simulink model "LQR_ACC_research"  (R2024a)
settings: Solver=FixedStepAuto  StartTime=0  StopTime=100  FixedStep=0.05  RelTol=1e-3
undefined symbols (not defined in the file or in its folder): acc_max, acc_min, Defined, driver_set_speed, Ego, jerk_lim, K_derr, K_vh, Lane, matlabshared, rho, simStepSize, User
libraries: roadrunnerscenario x5, dsa_UDP_Blockset x2, autolibshared x1, drivingscenarioandsensors x1
settings Model: PacingRate=10  Creator=darkh  LastModifiedBy=darkh
settings DataIOCC: ReturnWorkspaceOutputsName=sltest_internal_rrSimulationOutputVariable
settings DebuggingCC: AlgebraicLoopMsg=none
settings RTWCC: GPUComputeCapability=3.5
settings ConfigComp: CovSaveName=sltest_covdata  CovMetricSettings=dcmwe  CovEnableCumulative=off  CovSaveSingleToWorkspaceVar=on  CovSaveOutputData=off

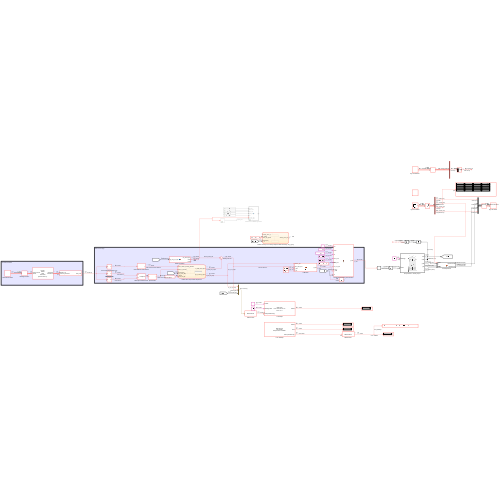
[thumbnail: Simulink's stored preview of the top-level diagram]
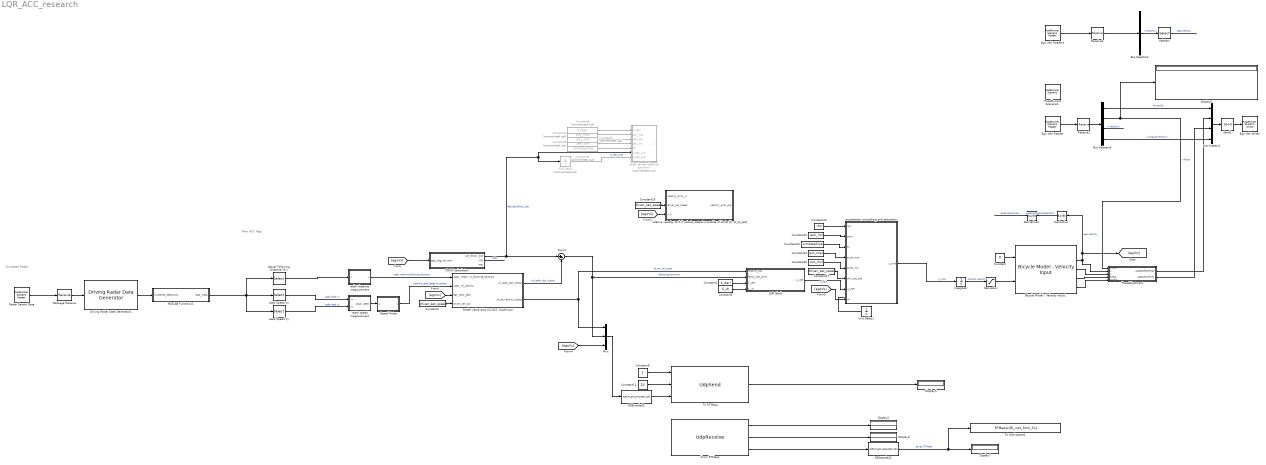
== system LQR_ACC_research ==
  note: Simulated Radar
  note: Main ACC Algo
  Actual Following Distance (dx) : Selector  InputPortWidth=6  IndexOptions=Index vector (dialog)  Indices=[1]  OutputSizes=1
  Bicycle Model - Velocity Input1 : autolibshared/Bicycle Model - Velocity Input  trackMode=Single (bicycle)  inputMode=External longitudinal velocity  frontSteerMode=on  rearSteerMode=off  windMode=off  muMode=off  extFMode=off  extMMode=off  aMode=3  NF=2  NR=2  m=2630.84  a=1.2  b=1.6  h=0.35  X_o=0  xdot_o=0  CalphaMode=off  sigmaMode=on  w=[1.4,1.4]  Cy_f=19000  Cy_r=33000  sigma_f=.1  sigma_r=.1  alpha_f_brk=[-.1 .1]  Cy_f_data=[-9e3 9e3]  alpha_r_brk=[-.1 .1]  Cy_r_data=[-9e3 9e3]  Y_o=0  ydot_o=0  Izz=2875  psi_o=0  r_o=0  Af=2  Cd=.3  Cl=.1  Cpm=.1  beta_w=[0 0.01:0.01:0.3]  Cs=[0 0.01:0.01:0.3]  Cym=[0 1e-6:0.01:0.3]  Pabs=101325  Tair=273  g=9.81  mu=1  xdot_tol=.01  Fznom=5000  Fxtire_sat=1e6  Fytire_sat=1e6  longOff=0  latOff=0  vertOff=0
      settings: LibrarySourceBlock=drivingscenarioandsensors/Bicycle Model - Velocity Input
  Bus Creator1 : BusCreator  Inputs=4  OutDataTypeStr=Bus: BusActorRuntime  NonVirtualBus=on
      settings: InheritFromInputs=off
  Bus Selector1 : BusSelector  OutputSignals=ActorRuntime.Velocity
  Bus Selector3 : BusSelector  OutputSignals=ActorID,Pose,Velocity,AngularVelocity
  Constant : Constant  Value=0
  Constant1 : Constant  Value=K_derr  SampleTime=simStepSize
  Constant10 : Constant  Value=rho
  Constant11 : Constant  Value=24
  Constant12 : Constant  Value=jerk_lim
  Constant13 : Constant  Value=simStepSize
  Constant14 : Constant  Value=acc_max
  Constant15 : Constant  Value=acc_min
  Constant16 : Constant  Value=driver_set_speed  SampleTime=simStepSize
  Constant17 : Constant  Value=driver_set_speed  SampleTime=simStepSize
  Constant2 : Constant  Value=driver_set_speed  SampleTime=simStepSize
  Constant3 : Constant  Value=K_vh  SampleTime=simStepSize
  Constant4 : Constant  Commented=on  Value=simStepSize
  Constant5 : Constant  Commented=on  Value=jerk_lim
  Constant6 : Constant  Commented=on  Value=acc_min
  Constant7 : Constant  Commented=on  Value=acc_max
  Constant8 : Constant  Commented=on  Value=K_derr
  Constant9 : Constant
  "DSDecode32 " : S-Function  FunctionName=ds867c_eth_decode32_sfcn  Parameters=byteordering,offset,auto_offset,datatype,one_datatype,sampletime  SFunctionDeploymentMode=off  EnableBusSupport=off  mask(DSDecode32){byteordering=big endian (Motorola), offset=[0], auto_offset=on, datatype=[9], one_datatype=off, sampletime=-1}
      mask prompts: byteordering "Byte ordering:"; offset "Offset (bytes):"; auto_offset "Auto offset"; one_datatype "One datatype only"
      mask help:
      | Converts a 32bit WORD input data stream into the specified datatypes on the output port.
      |
      | Datatype Codes:
      | BOOLEAN:  1   //   INT8      :  2    //   UINT8    :  3
      | INT16       :  4   //   UINT16 :  5    //   INT32     :  6
      | UINT32    :  7   //   FLOAT   :  8    //   DOUBLE:  9
      mask Help:
      | The 'DSDecode32' block allows to decode an UInt32 vector containing encoded elements of various data types to an output vector of double values. It is intended to use this block in conjunction with the 'DS4504_ETH_Receive' block which delivers this format as data output. Data received from the Ethernet via the 'DS4504_ETH_Receive' block is performed in Intel byte order ('Little Endian').
      | 
      | <br>
      | <br>
      | 
      | <h2>Parameters</h2>
      | <br>
      | <br>
      | 
      | <b>Byte ordering (only relevant for offline simulation)</b>
      | <br>
      | <blockquote>
      | The byte order of the input vector has to be specified. In case of running a real-time application the appropriate byte order (Motorola for DS1005 and Intel for DS1006) is selected automatically. Therefore the byte order setting has no influence on the online simulation.
      | </blockquote>
      | <br>
      | 
      | <b>Offset (bytes)</b>
      | <br>
      | <blockquote>
      | This is for defining a vector of offsets which specifies the position of each element within the input vector. The offsets must be entered as an array (e.g. [1 10 . 50 54] ) using the same order as for the corresponding data type vector (see (4)). This option is useful if you have gaps between adjacent elements.
      | </blockquote>
      | <br>
      | 
      | <b>Auto offset</b>
      | <br>
      | <blockquote>
      | When activating this checkbox parameter, the edit field 'Offset' is disabled and the byte offsets in the input vector are calculated automatically concerning the specified data types (no gaps presupposed). Any previous setting in the offset vector would be ignored.
      | </blockquote>
      | <br>
      | 
      | <b>Datatype</b>
      | <br>
      | <blockquote>
      | This is for defining a vector of data types which specifies the type for each element in the input vector. Supported data types are Boolean, Int8, UInt8, Int16, UInt16, Int32, UInt32, Float and Double, which are determined by using the corresponding data type codes shown in the following table:
      | <br>
      | <br>
      | <table BORDER=1 ALIGN="center">
      | <TR>
      | <TH WIDTH=20%>Data type</TH>
      | <TH WIDTH=20%>Data type code</TH>
      | <TH WIDTH=20%>Length in bytes</TH>
      | </TR>
      | <TR><TD>Boolean</TD><TD ALIGN="center">1</TD><TD ALIGN="center">1</TD></TR>
      | <TR><TD>Int8</TD><TD ALIGN="center">2</TD><TD ALIGN="center">1</TD></TR>
      | <TR><TD>Uint8</TD><TD ALIGN="center">3</TD><TD ALIGN="center">1</TD></TR>
      | <TR><TD>Int16</TD><TD ALIGN="center">4</TD><TD ALIGN="center">2</TD></TR>
      | <TR><TD>Uint16</TD><TD ALIGN="center">5</TD><TD ALIGN="center">2</TD></TR>
      | <TR><TD>Int32</TD><TD ALIGN="center">6</TD><TD ALIGN="center">4</TD></TR>
      | <TR><TD>Uint32</TD><TD ALIGN="center">7</TD><TD ALIGN="center">4</TD></TR>
      | <TR><TD>Float</TD><TD ALIGN="center">8</TD><TD ALIGN="center">4</TD></TR>
      | <TR><TD>Double</TD><TD ALIGN="center">9</TD><TD ALIGN="center">8</TD></TR>
      | </TABLE>
      | </blockquote>
      | <br>
      | 
      | <b>One datatype only</b>
      | <br>
      | <blockquote>
      | This option is useful if all elements of the input vector have the same data type. If the checkbox is activated the first element of the data type vector specifies the data type to be used. In this case it is naturally sufficient to enter only one number which applies for the complete input vector.
      | </blockquote>
      | <br>
      | 
      | <b>Sample time</b>
      | <br>
      | <blockquote>
      | The desired sample time for this block has to be entered here. Alternatively it can be  inherited from the Simulink model by using '-1'.
      | </blockquote>
      | <br>
      mask TypeOptions byteordering: big endian (Motorola) | little endian (Intel)
      mask Display: text(0.5,0.5,'DSDecode32','HorizontalAlignment','center')
  DSEncode32 : S-Function  FunctionName=ds867c_eth_encode32_sfcn  Parameters=byteordering,offset,auto_offset,datatype,one_datatype,sampletime  SFunctionDeploymentMode=off  EnableBusSupport=off  mask(DSEncode32){byteordering=big endian (Motorola), offset=[ 0 ], auto_offset=on, datatype=[9,9,9], one_datatype=off, sampletime=-1}
      mask prompts: byteordering "Byte ordering:"; offset "Offset (bytes):"; auto_offset "Auto offset"; one_datatype "One datatype only"
      mask help:
      | Converts an input signal consisting of datatypes into a 32Bit WORD data stream on the output port.
      |
      | Datatype Codes:
      | BOOLEAN:  1   //   INT8      :  2    //   UINT8    :  3
      | INT16       :  4   //   UINT16 :  5    //   INT32     :  6
      | UINT32    :  7   //   FLOAT   :  8    //   DOUBLE:  9
      mask Help:
      | The 'DSEncode32' block is responsible for converting the input vector consisting of double values to different data types (multi-byte numbers) and merging them into a data stream composed of an array of UInt32 variables. It is intended to use this block in conjunction with the 'DS4504_ETH_Send' block which delivers the data in Intel byte order to the network.
      | 
      | <br>
      | <br>
      | 
      | <h2>Parameters</h2>
      | <br>
      | <br>
      | 
      | <b>Byte ordering (only relevant for offline simulation)</b>
      | <br>
      | <blockquote>
      | It lets the user choose the byte order (Motorola or Intel) of the output vector. The way multibyte numbers (e.g. Float = 4 bytes or Int16 = 2 bytes) are stored in memory depends on the used computing system. There are two possible formats which are called "Little Endian" and "Big Endian". "Little Endian" means that the low-order byte of the number is stored at the lowest and the high-order byte at the highest memory address. "Big Endian" means the opposite.
      | This option is only relevant for offline (Simulink) simulation. In case of running a real-time application the appropriate byte order (Motorola for DS1005 and Intel for DS1006) is selected automatically. Therefore the byte order setting has no influence on the online simulation.
      | </blockquote>
      | <br>
      | 
      | <b>Offset (bytes)</b>
      | <br>
      | <blockquote>
      | This is for defining a vector of offsets which specifies the position of each input element within the output byte vector. The offsets must be entered as an array (e.g. [1 10 . 50 54] ) using the same order as for the corresponding data type vector (see (4)). This option is useful if you want to have gaps between adjacent elements (e.g. in order to avoid access to even bytes).
      | <br>
      | <br>
      | <i>Important Note:</i>
      | <br>
      | By means of the offset vector the specified data values can be located flexibly within the UInt32 word stream, presupposed that the data values do not overlap. Otherwise data loss occurs.
      | </blockquote>
      | <br>
      | 
      | <b>Auto offset</b>
      | <br>
      | <blockquote>
      | When activating this checkbox parameter, the edit field 'Offset' is disabled and the required byte offsets for the input data types will be calculated automatically without gaps (for tight packing). This option is always useful if there is no need for special offsets (no gaps between two adjacent elements). Any previous setting in the offset vector would be ignored.
      | </blockquote>
      | <br>
      | 
      | <b>Datatype</b>
      | <br>
      | <blockquote>
      | This is for defining a vector of data types which specifies the type for each input element in the output byte vector. Supported data types are Boolean, Int8, UInt8, Int16, UInt16, Int32, UInt32, Float and Double, which are determined by using the corresponding data type codes shown in the following table:
      | <br>
      | <br>
      | <table BORDER=1 ALIGN="center">
      | <TR>
      | <TH WIDTH=20%>Data type</TH>
      | <TH WIDTH=20%>Data type code</TH>
      | <TH WIDTH=20%>Length in bytes</TH>
      | </TR>
      | <TR><TD>Boolean</TD><TD ALIGN="center">1</TD><TD ALIGN="center">1</TD></TR>
      | <TR><TD>Int8</TD><TD ALIGN="center">2</TD><TD ALIGN="center">1</TD></TR>
      | <TR><TD>Uint8</TD><TD ALIGN="center">3</TD><TD ALIGN="center">1</TD></TR>
      | <TR><TD>Int16</TD><TD ALIGN="center">4</TD><TD ALIGN="center">2</TD></TR>
      | <TR><TD>Uint16</TD><TD ALIGN="center">5</TD><TD ALIGN="center">2</TD></TR>
      | <TR><TD>Int32</TD><TD ALIGN="center">6</TD><TD ALIGN="center">4</TD></TR>
      | <TR><TD>Uint32</TD><TD ALIGN="center">7</TD><TD ALIGN="center">4</TD></TR>
      | <TR><TD>Float</TD><TD ALIGN="center">8</TD><TD ALIGN="center">4</TD></TR>
      | <TR><TD>Double</TD><TD ALIGN="center">9</TD><TD ALIGN="center">8</TD></TR>
      | </TABLE>
      | </blockquote>
      | <br>
      | 
      | <b>One datatype only</b>
      | <br>
      | <blockquote>
      | This option is useful if all elements of the data input vector shall be converted to the same data type in the output vector. If the checkbox is activated the first element of the data type vector specifies the data type to be used. In this case it is naturally sufficient to enter only one number which applies for the complete input vector.
      | </blockquote>
      | <br>
      | 
      | <b>Sample time</b>
      | <br>
      | <blockquote>
      | The desired sample time for this block has to be entered here. Alternatively it can be  inherited from the Simulink model by using '-1'.
      | </blockquote>
      | <br>
      mask TypeOptions byteordering: big endian (Motorola) | little endian (Intel)
      mask Display: text(0.5,0.5,'DSEncode32','HorizontalAlignment','center')
  Derivative : Derivative
  Derivative1 : Derivative
  Display{2..3,5..7} (5 alike) : Display
  Driving Radar Data Generator1 : drivingscenarioandsensors/Driving Radar Data Generator  SensorIndex=1  UpdateRate=20  MountingLocation=[ 3.4, 0, 0.2 ]  MountingAngles=[0 0 0]  HasElevation=off  HasRangeRate=on  HasNoise=off  HasFalseAlarms=off  HasOcclusion=off  MaxNumReportsSource=Property  MaxNumReports=50  TargetReportFormat=Clustered detections  DetectionCoordinates=Body  TrackCoordinates=Body  BusNameSource=Auto  BusName=BusDrivingRadarDataGenerator  AzimuthResolution=4  ElevationResolution=5  RangeResolution=2.5  RangeRateResolution=0.05  AzimuthBiasFraction=0.1  ElevationBiasFraction=0.1  RangeBiasFraction=0.01  RangeRateBiasFraction=0.01  FieldOfView=[ 20, 5 ]  RangeLimits=[ 0, 150 ]  RangeRateLimits=[ -100, 100 ]  DetectionProbability=0.9  FalseAlarmRate=1e-06  ReferenceRange=100  ReferenceRCS=0  CenterFrequency=77e9  FilterInitializationFcn=initcvekf  ConfirmationThreshold=[2 3]  DeletionThreshold=[5 5]  InitialSeedSource=Repeatable  InitialSeed=0  UsedSeed=matlabshared.tracking.internal.SimulinkUtilities.seedManager(gcb)  ProfilesSource=From Scenario Reader block  ProfilesParameters=driving.internal.ActorProfilesRadarParameters  ProfilesExpression=struct('ClassID',0,'Length',4.7,'Width',1.8,'Height',1.4,'OriginOffset',[-1.35 0 0],'RCSPattern',[10 10;10 10],'RCSAzimuthAngles',[-180 180],'RCSElevationAngles',[-90 90])
  Ego Veh Reader : roadrunnerscenario/RoadRunner Scenario Reader  TopicCategory=Actor  ActorCategory=All Types  ActionType=Path Following  EventType=User-Defined  TopicType=Actor Pose  VehicleType=Vehicle Specifications  UserDefinedAction=Action1  UserDefinedEvent=Event1  Filter=Self  SensorTopic=Target Poses  LaneBoundaryOutputTopic=Ego-Lane  SensorID=1  SampleTime=simStepSize
  Ego Veh Reader1 : roadrunnerscenario/RoadRunner Scenario Reader  TopicCategory=Actor  ActorCategory=Vehicle  ActionType=Path Following  EventType=User-Defined  TopicType=Actor Pose  VehicleType=Vehicle Pose  UserDefinedAction=Action1  UserDefinedEvent=Event1  Filter=None  SensorTopic=Target Poses  LaneBoundaryOutputTopic=Ego-Lane  SensorID=1  SampleTime=simStepSize
  Ego Veh Writer : roadrunnerscenario/RoadRunner Scenario Writer  TopicCategory=Actor  ActorCategory=All Types  EventType=Action Complete  UserDefinedEvent=Event1  VehicleType=Vehicle Pose  TopicType=Actor Pose
  FDCW calculation : MATLAB Function  TreatAsAtomicUnit=on
  From RTMaps : dsa_UDP_Blockset/UdpReceive  portNumber=25000  sampleTime=simStepSize  outputWidth=1472  rxTimeout=1  rxBufferSize=73600
  Integrator : Integrator
  LQR Block : MATLAB Function  TreatAsAtomicUnit=on  SystemSampleTime=simStepSize
  Lead Speed Vx : Selector  InputPortWidth=6  IndexOptions=Index vector (dialog)  Indices=4  OutputSizes=1
  Lead Speed Vy : Selector  InputPortWidth=6  IndexOptions=Index vector (dialog)  Indices=5  OutputSizes=1
  MATLAB Function11 : MATLAB Function  TreatAsAtomicUnit=on
  Message Receive : Receive  InputPortMessageModes=m  UseInternalQueue=off
  Mux : Mux  Inputs=3
  PoseAdjustment : MATLAB Function  TreatAsAtomicUnit=on
  Radar Sensor Data : roadrunnerscenario/RoadRunner Scenario Reader  TopicCategory=Sensor  ActorCategory=All Types  ActionType=Path Following  EventType=User-Defined  TopicType=Actor Specifications  VehicleType=Vehicle Specifications  UserDefinedAction=Action1  UserDefinedEvent=Event1  Filter=Self  SensorTopic=Target Poses  LaneBoundaryOutputTopic=Ego-Lane  SensorID=1  SampleTime=simStepSize
  Radar value drop CC/ACC Supervisor : Stateflow chart  TreatAsAtomicUnit=on
  Receive1 : Receive  InputPortMessageModes=m  UseInternalQueue=off  QueueOverwriting=on  QueueLength=1  QueueType=LIFO
  Receive2 : Receive  InputPortMessageModes=m  UseInternalQueue=off  QueueOverwriting=on  QueueLength=1  QueueType=LIFO
  RoadRunner Scenario1 : roadrunnerscenario/RoadRunner Scenario  UserDefinedActions={}  UserDefinedEvents={}
  Saturation : Saturate  UpperLimit=driver_set_speed  LowerLimit=0
  Selector : Selector  InputPortWidth=3  IndexOptions=Index vector (dialog)  Indices=[1]  OutputSizes=1
  Send1 : Send  OutputPortMessageModes=m
  Speed Noise : MATLAB Function  TreatAsAtomicUnit=on
  Sum4 : Sum  Inputs=|+-
  To RTMaps : dsa_UDP_Blockset/UdpSend  hostName=192.168.140.10  portNumber=11111
  To Workspace1 : ToWorkspace  VariableName=RTMapsLQR_inpt_from_SL1  SaveFormat=Timeseries  SampleTime=-1
  Unit Delay : UnitDelay  Commented=on  SampleTime=-1  HasFrameUpgradeWarning=on
  Unit Delay1 : UnitDelay  SampleTime=-1  HasFrameUpgradeWarning=on
  acceleration smoothing and saturation : MATLAB Function  TreatAsAtomicUnit=on  SystemSampleTime=simStepSize
  delta desired distance governor : MATLAB Function  Commented=on  TreatAsAtomicUnit=on
  radar distance measurement : MATLAB Function  TreatAsAtomicUnit=on
  radar speed measurement : MATLAB Function  TreatAsAtomicUnit=on
  "relative velocity to 0 if velocity setpoint outside of limits [0, dr_st_spd]" : Stateflow chart  TreatAsAtomicUnit=on
  wires:
  Bus Selector3/4 -> Bus Creator1/4  "<AngularVelocity>"
  Bus Creator1/1 -> Send1/1
  Bus Selector3/1 -> Bus Creator1/1  "<ActorID>"
  Receive1/1 -> Bus Selector3/1
  Send1/1 -> Ego Veh Writer/1
  Ego Veh Reader/1 -> Receive1/1
  Bicycle Model - Velocity Input1/3 -> PoseAdjustment/3(v)
  Bicycle Model - Velocity Input1/4 -> PoseAdjustment/4(theta)
  Bicycle Model - Velocity Input1/5 -> PoseAdjustment/5(omega)
  Bus Selector3/2 -> Display6/1, PoseAdjustment/1(cPose)  "<Pose>"
  PoseAdjustment/1(updatedPoseMat) -> Bus Creator1/2
  Bicycle Model - Velocity Input1/2 -> Derivative/1, [egoVx], PoseAdjustment/2(u)  "ego velocity"
  Radar Sensor Data/1 -> Message Receive/1
  Message Receive/1 -> Driving Radar Data Generator1/1
  Driving Radar Data Generator1/1 -> MATLAB Function11/1(clustered_detections)
  PoseAdjustment/2(updatedVelVec) -> Bus Creator1/3
  Integrator/1 -> Saturation/1  "Control Velocity"
  Constant/1 -> Bicycle Model - Velocity Input1/1
  Sum4/1 -> Mux/2, LQR Block/2(follow_dist_error)  "following dist error"
  Constant1/1 -> LQR Block/3(K_derr)
  Lead Speed Vx/1 -> radar speed measurement/1(Vx)  "radar lead Vx"
  [egoVx] -> FDCW calculation/1(ego_long_vel_mph)
  FDCW calculation/1(ave_follow_dist) -> Sum4/1, delta desired distance governor/6(d_des_curr), Unit Delay/1  "desired_follow_dist"
  MATLAB Function11/1(lead_meas) -> Actual Following Distance (dx)/1, Lead Speed Vy/1, Lead Speed Vx/1
  Lead Speed Vy/1 -> radar speed measurement/2(Vy)  "radar lead Vy"
  radar speed measurement/1(LeadSpeed) -> Speed Noise/1(u)
  FDCW calculation/2(CFD) -> ?  "CFD"
  Actual Following Distance (dx)/1 -> radar distance measurement/1(u)
  Derivative/1 -> Derivative1/1  "experienced acceleration"
  Derivative1/1 -> ?  "experienced jerk"
  [egoVx] -> Radar value drop CC/ACC Supervisor/3(ego_veloc_fdbk)
  Constant2/1 -> Radar value drop CC/ACC Supervisor/4(driver_set_spd)
  Speed Noise/1(y) -> Radar value drop CC/ACC Supervisor/2(radar_rel_velocity)  "relative Lead Speed no spikes"
  radar distance measurement/1(y) -> Radar value drop CC/ACC Supervisor/1(radar_relative_following_distance)  "radar relative following distance"
  Radar value drop CC/ACC Supervisor/1(sf_radar_dist_output) -> Sum4/2  "sf_radar_dist_output"
  Radar value drop CC/ACC Supervisor/2(sf_rel_velocity_output) -> LQR Block/1(relative_spd), Mux/1  "sf_rel_vel_outpt"
  Constant3/1 -> LQR Block/4(K_vh)
  Unit Delay/1 -> delta desired distance governor/7(d_des_prev)  "d_des_prev"
  Constant4/1 -> delta desired distance governor/5(Ts)
  Constant5/1 -> delta desired distance governor/4(jerk_lim)
  Constant6/1 -> delta desired distance governor/3(acc_min)
  Constant7/1 -> delta desired distance governor/2(acc_max)
  Constant8/1 -> delta desired distance governor/1(K_derr)
  Mux/1 -> DSEncode32/1
  Constant9/1 -> To RTMaps/1
  Constant11/1 -> To RTMaps/2
  To RTMaps/1 -> Display5/1
  From RTMaps/1 -> Display2/1
  From RTMaps/2 -> Display3/1
  From RTMaps/3 -> "DSDecode32 "/1
  DSEncode32/1 -> To RTMaps/3
  "DSDecode32 "/1 -> Display7/1, To Workspace1/1  "accel_RTMaps"
  LQR Block/1(u_LQR) -> acceleration smoothing and saturation/7(u_LQR)  "u_LQR"
  Constant12/1 -> acceleration smoothing and saturation/2(Jmax)
  Constant13/1 -> acceleration smoothing and saturation/3(Ts)
  Constant14/1 -> acceleration smoothing and saturation/4(accel_max)
  Constant15/1 -> acceleration smoothing and saturation/5(accel_min)
  Unit Delay1/1 -> ?
  Constant10/1 -> acceleration smoothing and saturation/1(rho)
  Constant16/1 -> "relative velocity to 0 if velocity setpoint outside of limits [0, dr_st_spd]"/2(driver_set_speed)
  [egoVx] -> "relative velocity to 0 if velocity setpoint outside of limits [0, dr_st_spd]"/3(v_h)
  [egoVx] -> acceleration smoothing and saturation/8(vh)
  Constant17/1 -> acceleration smoothing and saturation/6(drvr_set_spd)
  Ego Veh Reader1/1 -> Receive2/1
  Receive2/1 -> Bus Selector1/1
  Bus Selector1/1 -> Selector/1  "<Velocity>"
  Bus Selector3/3 -> ?  "<Velocity>"
  Selector/1 -> ?  "lead velocity"
  Saturation/1 -> Bicycle Model - Velocity Input1/2
  [egoVx] -> Mux/3
  acceleration smoothing and saturation/1(u_cmd) -> Integrator/1  "u_cmd"

== matlab function LQR_ACC_research/PoseAdjustment ==
  data: cPose input; u input; updatedPoseMat output; v input; theta input; omega input; updatedVelVec output
function [updatedPoseMat, updatedVelVec] = fcn(cPose, u, v, theta, omega)
    thetad = theta + omega*(1/10)
    xd = (u*cos(theta) - v*sin(theta))*(1/10)
    yd = (u*sin(theta) + v*cos(theta))*(1/10)
    pose_mat = [cos(-thetad) -sin(-thetad) 0 (yd+cPose(1,4)); sin(-thetad) cos(-thetad) 0 (xd+cPose(2,4)); 0 0 1 0; 0 0 0 1];
    updatedPoseMat = pose_mat;
    updatedVelVec = [u*sin(theta) + v*cos(theta), u*cos(theta) - v*sin(theta), 0];
    return;
end

== matlab function LQR_ACC_research/radar distance measurement ==
  data: u input; y output
function y = removeSpikes(u)

    persistent buffer;
    persistent bufferIndex;
    threshold = 2;
    windowSize = 15;
    % windowSize = 4;
    
    if isempty(buffer)
        buffer = zeros(1, windowSize);
        bufferIndex = 1;
    end
    
    % Update buffer with new value
    buffer(bufferIndex) = u;
    bufferIndex = mod(bufferIndex, windowSize) + 1;
    
    % Calculate the median of the buffer
    medVal = median(buffer);
    
    % Detect and remove spikes
    if abs(u - medVal) > threshold
        y = medVal; % Replace spike with the median value
    else
        y = u; % Keep the original value if it's not a spike
    end
end

== matlab function LQR_ACC_research/radar speed measurement ==
  data: Vx input; LeadSpeed output; Vy input
function LeadSpeed = fcn(Vx, Vy)

if Vx == 0 && Vy == 0 
    Vx = 0.01;
    Vy = 0.01;
elseif Vy == 0
    Vy = 0.01;
elseif Vx == 0
    Vx = 0.01;
end

if Vx <= 0
    LeadSpeed = -sqrt(Vx^2 + Vy^2);
else
    LeadSpeed = sqrt(Vx^2 + Vy^2);
end

== matlab function LQR_ACC_research/Speed Noise ==
  settings: updateMethod=DISCRETE
  data: u input; y output
function y = removeSpikes(u)
    % removeSpikes - Removes spikes from a scalar signal based on a threshold
    %
    % Inputs:
    %    u - The input signal (scalar)
    %    threshold - The threshold value to detect spikes
    %    windowSize - The size of the window for calculating the median
    %
    % Outputs:
    %    y - The filtered signal with spikes removed

    % Declare persistent variables to store past values
    persistent buffer;
    persistent bufferIndex;
    threshold = 2;
    windowSize = 15;
    % windowSize = 5;

    
    if isempty(buffer)
        buffer = zeros(1, windowSize);
        bufferIndex = 1;
    end
    
    % Update buffer with new value
    buffer(bufferIndex) = u;
    bufferIndex = mod(bufferIndex, windowSize) + 1;
    
    % Calculate the median of the buffer
    medVal = median(buffer);
    
    % Detect and remove spikes
    if abs(u - medVal) > threshold
        y = medVal; % Replace spike with the median value
    else
        y = u; % Keep the original value if it's not a spike
    end
end

== matlab function LQR_ACC_research/MATLAB Function11 ==
  data: clustered_detections input Bus: BusRadar; lead_meas output double
function lead_meas = fcn(clustered_detections)

lead_det = clustered_detections.Detections(1);
lead_meas = lead_det.Measurement;

% relative_dist = sqrt(lead_det.Measurement(1)^2 + lead_det.Measurement(2)^2); % rel_dist = sqrt(x^2+y^2)
% relative_speed = sqrt(lead_det.Measurement(4)^2 + lead_det.Measurement(5)^2);
end

== matlab function LQR_ACC_research/FDCW calculation ==
  settings: updateMethod=DISCRETE
  data: ego_long_vel_mph input; ave_follow_dist output; CFD output; FFD output
% Function to determine the closest (CFD) and furthest follow distance (FFD) for the
% ego vehicle relative to the lead vehicle given the ego vehicle's current
% velocity

% This function outputs the middle distance value between the CFD and FFD
% and those values respectively as well

function [ave_follow_dist, CFD, FFD] = fcn(ego_long_vel_mph)
    persistent dist_history window_size smoothing_weights
    
    % Initialize (first call only)
    if isempty(dist_history)
        window_size = 5;  % Number of past samples
        dist_history = zeros(1, window_size);
        
        % Define and normalize weights (e.g., linear decay)
        smoothing_weights = linspace(1, 0.5, window_size);  % Weights from 1.0 to 0.5
        smoothing_weights = smoothing_weights / sum(smoothing_weights);  % Normalize
    end

    if ego_long_vel_mph > 0 && ego_long_vel_mph < 20
        CFD = 2.8*ego_long_vel_mph^0.45+8;
        FFD = 100-0.2*(20-ego_long_vel_mph)^2;
    elseif ego_long_vel_mph <= 0
        CFD = 8;
        FFD = 100-0.2*(20)^2;
    else
        CFD = 2.8*ego_long_vel_mph^0.45+8;
        FFD = 100;
    end
    AveFollowDist_Gain = 2;


    % --- Update history buffer ---
    dist_history = [ ((AveFollowDist_Gain-1)*CFD + FFD)/AveFollowDist_Gain , dist_history(1:end-1)];  % FIFO

    % --- Smoothed average (weighted, normalized) ---
    smoothed_ave_dist = sum(dist_history .* smoothing_weights);
    
    % --- Clamp to CFD/FFD bounds ---
    ave_follow_dist = min(max(smoothed_ave_dist, CFD), FFD);
end

== matlab function LQR_ACC_research/LQR Block ==
  data: relative_spd input; u_LQR output; follow_dist_error input; K_derr input; K_vh input
function u_LQR = fcn(relative_spd, follow_dist_error, K_derr, K_vh)
u_LQR = -K_derr*follow_dist_error-K_vh*relative_spd;

== matlab function LQR_ACC_research/delta desired distance governor ==
  data: K_derr input; y output; acc_max input; acc_min input; jerk_lim input; Ts input; d_des_curr input; d_des_prev input
function y = fcn(K_derr, acc_max, acc_min, jerk_lim, Ts, d_des_curr, d_des_prev)

y = u;

== stateflow chart LQR_ACC_research/Radar value drop CC//ACC Supervisor ==
  state Radar_State_Lead_Veh_Present_and_Detected
    sf_radar_dist_output = radar_relative_following_distance;
    sf_rel_velocity_output = radar_rel_velocity;
    counter = counter + 1; % updates by 1 every time step; to wait to give the radar time to initialize in simulation
  state Output_Spoof_To_Keep_Moving
    %sf_radar_dist_output = 150;
    sf_radar_dist_output = smooth_switch(sf_radar_dist_output, 70, 0.05, 2);
    set_spd_err = driver_set_spd - ego_veloc_fdbk;
    sf_rel_velocity_output = set_spd_err;
    % sf_rel_velocity_output = smooth_switch(sf_rel_velocity_output, set_spd_err, 0.05, 5);
  (default) -> Radar_State_Lead_Veh_Present_and_Detected : {sf_radar_dist_output = radar_relative_following_distance;
      | sf_rel_velocity_output = radar_rel_velocity;
      | counter = 0;}
  Radar_State_Lead_Veh_Present_and_Detected -> Output_Spoof_To_Keep_Moving : [radar_relative_following_distance == 0 && radar_rel_velocity < 0.9 && counter > 20]
  Output_Spoof_To_Keep_Moving -> Radar_State_Lead_Veh_Present_and_Detected : [radar_relative_following_distance > 0]
  data: prev_val function_input; curr_val function_input; dt function_input; tau function_input; filtered_val function_output; radar_relative_following_distance input; sf_radar_dist_output output; radar_rel_velocity input; ego_veloc_fdbk input; sf_rel_velocity_output output; driver_set_spd input; set_spd_err local; counter local
  function filtered_val = smooth_switch(prev_val, curr_val, dt, tau):
    | function filtered_val = smooth_switch(prev_val, curr_val, dt, tau)
    | % Smooth transition from prev_val toward curr_val
    | % dt  = sample time [s]; equal to system sample time of 0.05s currently
    | % tau = time constant [s] (0.3–1.0 typical)
    | 
    | if isempty(prev_val)
    |     prev_val = 0;
    | end
    | 
    | alpha = exp(-dt/tau);
    | filtered_val = alpha*prev_val + (1-alpha)*curr_val;
    | end

== matlab function LQR_ACC_research/acceleration smoothing and saturation ==
  data: rho input; Jmax input; Ts input; accel_max input; accel_min input; drvr_set_spd input; u_cmd output; u_LQR input; vh input
function u_cmd = fcn(rho, Jmax, Ts, accel_max, accel_min, drvr_set_spd, u_LQR, vh) % ,u_k_minus_1)
% This function is the smoothing step that determines a commanded control
% signal based on minimizing the following QP : J(u) = (u-u_lqr)^2 + rho*(u - uk_minus_1)^2

persistent u_k_minus_1
if isempty(u_k_minus_1)
    u_k_minus_1 = 0.0;
end

u_tilde = (u_LQR + rho*u_k_minus_1)/(1 + rho);

u_cmd = min(max(u_tilde, u_k_minus_1 - Jmax*Ts), u_k_minus_1 + Jmax*Ts); % rate-limiting the control signal (jerk limits)
u_cmd = min(max(u_cmd, accel_min), accel_max); % Applying acceleration magnitude limits to control signal
u_k_minus_1 = u_cmd; % updating previous input value for use next timestep

if (vh <= 0.001 && u_cmd < 0.0) % If vehicle is at a full stop and controller requests a negative acceleration, set commanded accel to 0 m/s^2
    u_cmd = 0.0;
    u_k_minus_1 = u_cmd; % updating previous input value for use next timestep

elseif (vh >= drvr_set_spd && u_cmd > 0.0) % If vehicle is at driver set limit and controller requests positive accel, set command to 0 m/s^2
    % filtered_val = alpha*prev_val + (1-alpha)*curr_val; Smooth transition from prev_val toward curr_val; where alpha = exp(-dt/tau)
    % dt  = sample time [s]; equal to system sample time of 0.05s currently
    % tau = time constant [s] (0.3–1.0 typical)
    alpha = exp(-Ts/0.5);
    u_cmd = alpha*u_k_minus_1 + (1-alpha)*0.0;
    % u_cmd = 0.0;
    u_k_minus_1 = u_cmd; % updating previous input value for use next timestep
end

== stateflow chart LQR_ACC_research/relative velocity to 0 if velocity setpoint outside of limits [0, dr_st_spd] ==
  state relay_relative_velocity_as_is
    velocity_error_out = velocity_error_in;
    velocity_setpoint = v_h + velocity_error_in;
  state saturate_relative_velocity_error
    velocity_error_out = 0.0;
  (default) -> relay_relative_velocity_as_is
  relay_relative_velocity_as_is -> saturate_relative_velocity_error : [velocity_setpoint < 0.0 || velocity_setpoint > driver_set_speed]
  data: velocity_error_in input; velocity_error_out output; driver_set_speed input; v_h input; velocity_setpoint local
